simulink model "InverseKin"  (R2020b)
settings: Solver=VariableStepAuto  StartTime=0.0  StopTime=10.0  RelTol=1e-3
settings Model: Creator=b  LastModifiedBy=b

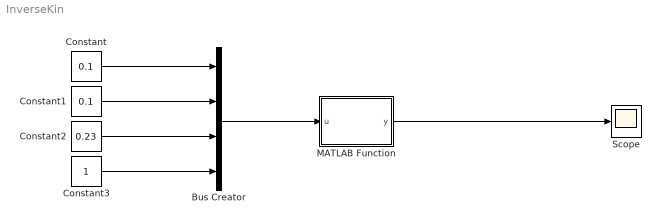
== system InverseKin ==
  Bus Creator : BusCreator  Inputs=4
  Constant : Constant  Value=0.1
  Constant1 : Constant  Value=0.1
  Constant2 : Constant  Value=0.23
  Constant3 : Constant
  MATLAB Function : MATLAB Function  TreatAsAtomicUnit=on
  Scope : Scope
  wires:
  Constant/1 -> Bus Creator/1
  Constant1/1 -> Bus Creator/2
  Constant2/1 -> Bus Creator/3
  Constant3/1 -> Bus Creator/4
  Bus Creator/1 -> MATLAB Function/1(u)
  MATLAB Function/1(y) -> Scope/1

== matlab function InverseKin/MATLAB Function ==
  data: u input; y output
function y = fcn(u)
d1 = 0.23500;
d2 = 0.21675;
d3 = 0.10875;
%d4 = 0.03000;

%u = [d2+d3-0.01;0;d1;0];
x = u(1);
y = u(2);
z = u(3);
pitch = u(4);

r = sqrt(x^2+y^2+(z-d1)^2)
theta1 = atan2(y,x)
theta2 = atan((z-d1)/sqrt(x^2+y^2)) + acos((d2^2+r^2-d3^2)/(2*d2*r))
theta3 = acos((d2^2 + d3^2 - r^2) / (2 * d2 * d3))
theta4 = theta2+theta3-pitch
q = [theta1;theta2;theta3;theta4];
y = q
